simulink model "Question4"  (R2020a)
settings: Solver=VariableStepAuto  StartTime=0.0  StopTime=10.0  RelTol=1e-3
model workspace (MAT data in the model file):
  J = Simulink.Parameter
  J.Value = 80
  J.DataType = 'auto'
  J.Dimensions = [1 1]
  K = Simulink.Parameter
  K.Value = 200
  K.DataType = 'auto'
  K.Dimensions = [1 1]
  Kd = Simulink.Parameter
  Kd.Value = 0.01
  Kd.DataType = 'auto'
  Kd.Dimensions = [1 1]
  Ki = Simulink.Parameter
  Ki.Value = 50
  Ki.DataType = 'auto'
  Ki.Dimensions = [1 1]
  Kp = Simulink.Parameter
  Kp.Value = 100
  Kp.DataType = 'auto'
  Kp.Dimensions = [1 1]
  L = Simulink.Parameter
  L.Value = 60
  L.DataType = 'auto'
  L.Dimensions = [1 1]
  R = Simulink.Parameter
  R.Value = 30
  R.DataType = 'auto'
  R.Dimensions = [1 1]
  b = Simulink.Parameter
  b.Value = 50
  b.DataType = 'auto'
  b.Dimensions = [1 1]
settings Model: OrderedModelArguments=off  Creator=anjal  LastModifiedBy=anjal

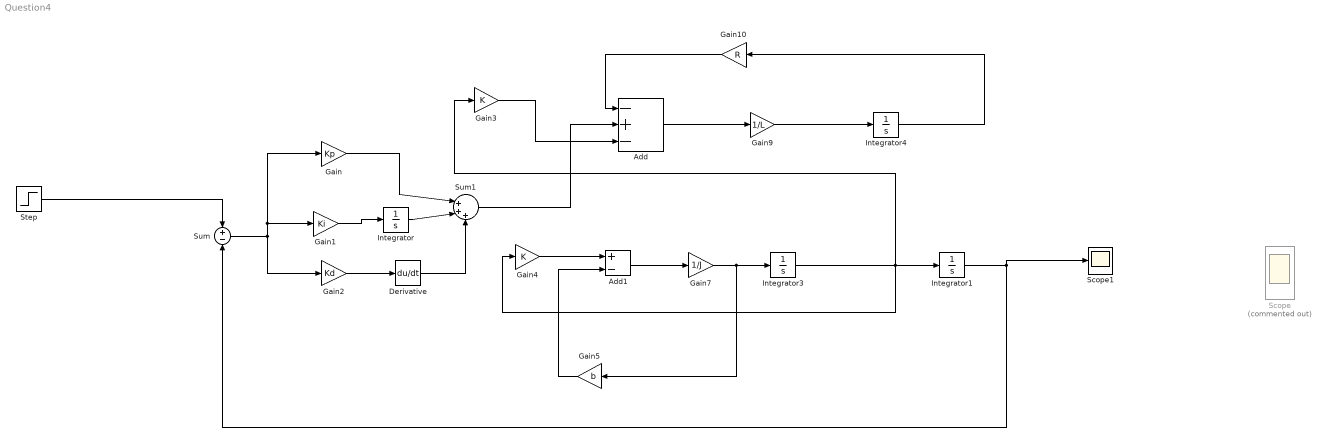
== system Question4 ==
  Add : Sum  Inputs=-+-
  Add1 : Sum  Inputs=+-
  Derivative : Derivative
  Gain : Gain  Gain=Kp
  Gain1 : Gain  Gain=Ki
  Gain10 : Gain  Gain=R
  Gain2 : Gain  Gain=Kd
  Gain3 : Gain  Gain=K
  Gain4 : Gain  Gain=K
  Gain5 : Gain  Gain=b
  Gain7 : Gain  Gain=1/J
  Gain9 : Gain  Gain=1/L
  Integrator{,1,3..4} (4 alike) : Integrator
  Scope : Scope  Commented=on  NumInputPorts=2
  Scope1 : Scope
  Step : Step  SampleTime=0
  Sum : Sum  Inputs=+-
  Sum1 : Sum  Inputs=|+++
  wires:
  Sum1/1 -> Add/2
  Gain9/1 -> Integrator4/1
  Gain1/1 -> Integrator/1
  Gain2/1 -> Derivative/1
  Add1/1 -> Gain7/1
  Gain/1 -> Sum1/1
  Step/1 -> Sum/1
  Sum/1 -> Gain2/1, Gain/1, Gain1/1
  Derivative/1 -> Sum1/3
  Integrator4/1 -> Gain10/1
  Gain5/1 -> Add1/2
  Gain4/1 -> Add1/1
  Integrator3/1 -> Integrator1/1, Gain3/1, Gain4/1
  Gain10/1 -> Add/1
  Integrator1/1 -> Sum/2, Scope1/1
  Gain3/1 -> Add/3
  Integrator/1 -> Sum1/2
  Gain7/1 -> Gain5/1, Integrator3/1
  Add/1 -> Gain9/1
